simulink model "Simulink_Lab_06"  (R2023a)
settings: Solver=VariableStepAuto  StartTime=0.0  StopTime=4  RelTol=1e-3
undefined symbols (not defined in the file): A, B, C, D, x0
settings Model: Creator=Mawuse  LastModifiedBy=Mawuse

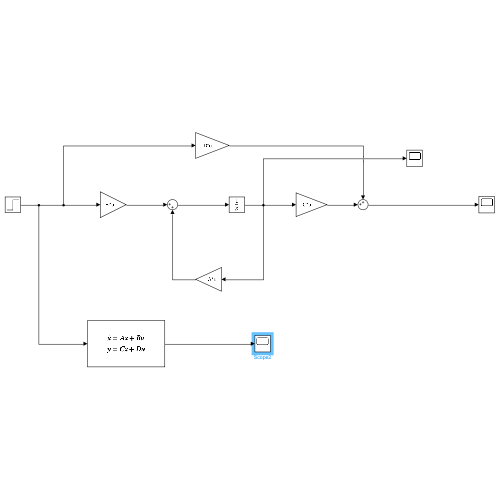
[thumbnail: Simulink's stored preview of the top-level diagram]
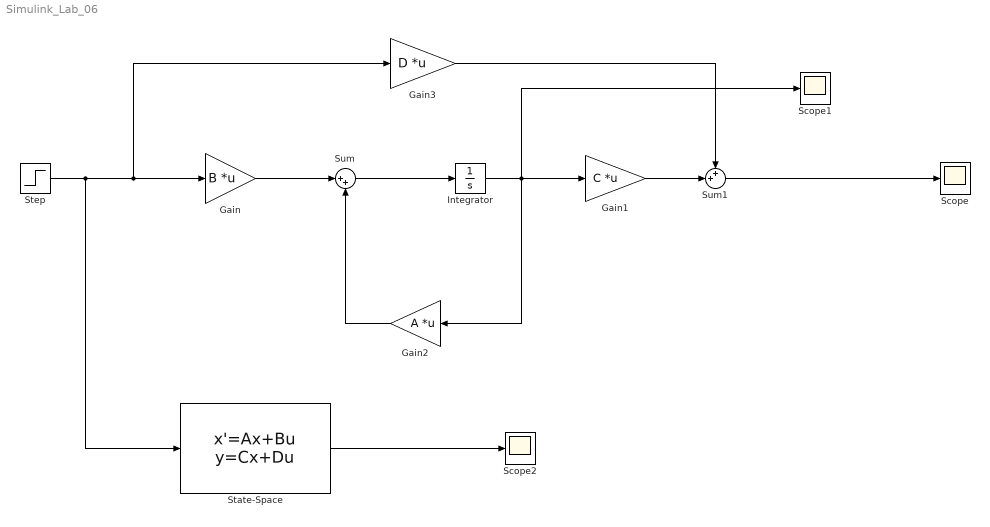
== system Simulink_Lab_06 ==
  Gain : Gain  Gain=B  Multiplication=Matrix(K*u)
  Gain1 : Gain  Gain=C  Multiplication=Matrix(K*u)
  Gain2 : Gain  Gain=A  Multiplication=Matrix(K*u)
  Gain3 : Gain  Gain=D  Multiplication=Matrix(K*u)
  Integrator : Integrator  InitialCondition=x0
  Scope : Scope
  Scope1 : Scope
  Scope2 : Scope
  State-Space : StateSpace  A=A  B=B  C=C  D=D  InitialCondition=x0  ParameterTunability=Unconstrained
  Step : Step  Time=0  SampleTime=0
  Sum : Sum  Inputs=|++
  Sum1 : Sum  Inputs=++|
  wires:
  Step/1 -> State-Space/1, Gain3/1, Gain/1
  Gain/1 -> Sum/1
  Sum/1 -> Integrator/1
  Gain2/1 -> Sum/2
  Integrator/1 -> Scope1/1, Gain2/1, Gain1/1
  Gain3/1 -> Sum1/1
  Gain1/1 -> Sum1/2
  Sum1/1 -> Scope/1
  State-Space/1 -> Scope2/1
